simulink model "stabilization_loop"  (R2017a)
settings: Solver=ode4  StartTime=0.0  StopTime=1  FixedStep=0.001  RelTol=1e-3
values from neighbouring files (symbols this model uses):
  K = -a13 * a42 / (a11*a42 + a12)    [D_partition.m]
  T = 1 / sqrt(a11*a42 + a12)    [D_partition.m]
  T1 = 1 / a42    [D_partition.m]
libraries: checkpacklib x1
settings Model: Creator=Alex  LastModifiedBy=Alex

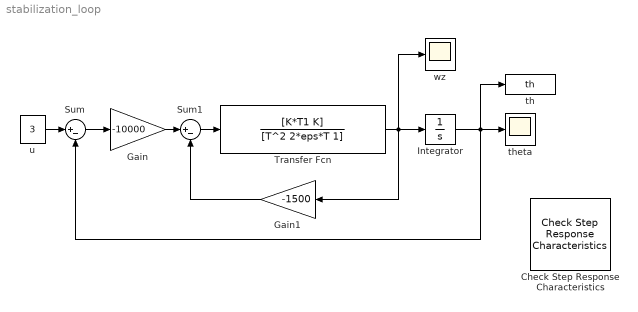
== system stabilization_loop ==
  Check Step Response Characteristics : checkpacklib/Check Step Response  Characteristics  InstantiateOnLoad=on  enabled=on  stopWhenAssertionFail=off  export=off  ViewDlgPos=[]  OpenViewOnLoad=off  LaunchViewOnOpen=off  TimeUnits=seconds  EnableStepResponseBound=on  InitialValue=0  FinalValue=3  StepTime=0  RiseTime=0.8  PercentRise=80  SettlingTime=1  PercentSettling=0  PercentOvershoot=0  PercentUndershoot=0
  Gain : Gain  Gain=-10000
  Gain1 : Gain  Gain=-1500
  Integrator : Integrator
  Sum : Sum  Inputs=|+-
  Sum1 : Sum  Inputs=|+-
  Transfer Fcn : TransferFcn  Numerator=[K*T1 K]  Denominator=[T^2 2*eps*T 1]
  th : ToWorkspace  VariableName=th  SaveFormat=Timeseries  SampleTime=-1
  theta : Scope
  u : Constant  Value=3
  wz : Scope
  wires:
  u/1 -> Sum/1
  Sum/1 -> Gain/1
  Gain/1 -> Sum1/1
  Sum1/1 -> Transfer Fcn/1
  Transfer Fcn/1 -> wz/1, Integrator/1, Gain1/1
  Integrator/1 -> th/1, theta/1, Sum/2
  Gain1/1 -> Sum1/2
